simulink model "ActiveBalancer20S"  (R2021a)
settings: Solver=VariableStepAuto  StartTime=0.0  StopTime=1500  RelTol=1e-3
undefined symbols (not defined in the file): Ion, Lithium
libraries: spsSeriesRLCBranchLib x38, spsIdealSwitchLib x22, spsBatteryLib x20, spsDiodeLib x20, spsCurrentMeasurementLib x1, spsDCVoltageSourceLib x1, spsGroundLib x1, spsPWMGenerator2LevelLib x1, spspowerguiLib x1
settings Model: SimulationMode=rapid-accelerator  Creator=jafar  LastModifiedBy=jafar

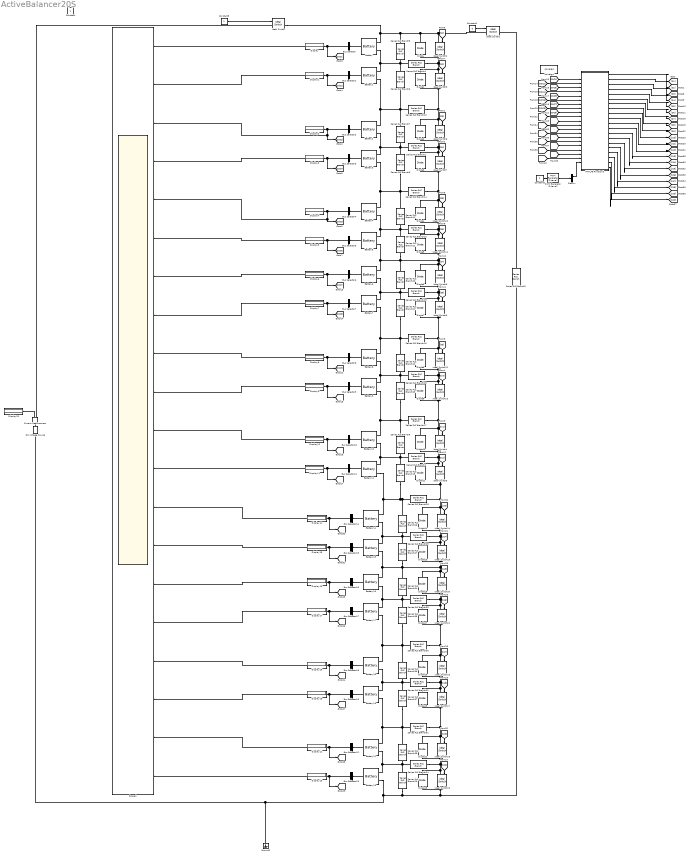
== system ActiveBalancer20S ==
  Battery : spsBatteryLib/Battery  BatType=Lithium-Ion  ShowTempParam=off  ThermalPreset=no  ShowAgeParam=off  NomV=3.7  NomQ=30  SOC=20  Batt_Tr=30  PresetModel=on  MaxQ=30  MinV=2.775  FullV=4.3068  Dis_rate=13.0435  R=0.0012333  Normal_OP=27.1304  expZone="[3.9974      1.4739]"  current=[6.5 13 32.5]  Units=Time  Tci=20  NomT=20  T2=-30  MaxQ2=4.8  FullV2=7.1  Normal_OP2=5.655  expZone2="[6.58           1]"  Rca=0.6  ti=2000  Dp=0  Neq0=0  Tsim=1e6  Ta1=25  Qeol=5.4*0.9  Reol=0.013333*1.2  Char_age=[2.3478, 3]  Dis_age=[2.3478, 10]  N1=1500  N2=10500  N3=1000  N4=1400  Ta2=45  N5=950
  Battery1 : spsBatteryLib/Battery  BatType=Lithium-Ion  ShowTempParam=off  ThermalPreset=no  ShowAgeParam=off  NomV=3.7  NomQ=30  SOC=23  Batt_Tr=30  PresetModel=on  MaxQ=30  MinV=2.775  FullV=4.3068  Dis_rate=13.0435  R=0.0012333  Normal_OP=27.1304  expZone="[3.9974      1.4739]"  current=[6.5 13 32.5]  Units=Time  Tci=20  NomT=20  T2=-30  MaxQ2=4.8  FullV2=7.1  Normal_OP2=5.655  expZone2="[6.58           1]"  Rca=0.6  ti=2000  Dp=0  Neq0=0  Tsim=1e6  Ta1=25  Qeol=5.4*0.9  Reol=0.013333*1.2  Char_age=[2.3478, 3]  Dis_age=[2.3478, 10]  N1=1500  N2=10500  N3=1000  N4=1400  Ta2=45  N5=950
  Battery10 : spsBatteryLib/Battery  BatType=Lithium-Ion  ShowTempParam=off  ThermalPreset=no  ShowAgeParam=off  NomV=3.7  NomQ=30  SOC=60  Batt_Tr=30  PresetModel=on  MaxQ=30  MinV=2.775  FullV=4.3068  Dis_rate=13.0435  R=0.0012333  Normal_OP=27.1304  expZone="[3.9974      1.4739]"  current=[6.5 13 32.5]  Units=Time  Tci=20  NomT=20  T2=-30  MaxQ2=4.8  FullV2=7.1  Normal_OP2=5.655  expZone2="[6.58           1]"  Rca=0.6  ti=2000  Dp=0  Neq0=0  Tsim=1e6  Ta1=25  Qeol=5.4*0.9  Reol=0.013333*1.2  Char_age=[2.3478, 3]  Dis_age=[2.3478, 10]  N1=1500  N2=10500  N3=1000  N4=1400  Ta2=45  N5=950
  Battery11 : spsBatteryLib/Battery  BatType=Lithium-Ion  ShowTempParam=off  ThermalPreset=no  ShowAgeParam=off  NomV=3.7  NomQ=30  SOC=63  Batt_Tr=30  PresetModel=on  MaxQ=30  MinV=2.775  FullV=4.3068  Dis_rate=13.0435  R=0.0012333  Normal_OP=27.1304  expZone="[3.9974      1.4739]"  current=[6.5 13 32.5]  Units=Time  Tci=20  NomT=20  T2=-30  MaxQ2=4.8  FullV2=7.1  Normal_OP2=5.655  expZone2="[6.58           1]"  Rca=0.6  ti=2000  Dp=0  Neq0=0  Tsim=1e6  Ta1=25  Qeol=5.4*0.9  Reol=0.013333*1.2  Char_age=[2.3478, 3]  Dis_age=[2.3478, 10]  N1=1500  N2=10500  N3=1000  N4=1400  Ta2=45  N5=950
  Battery12 : spsBatteryLib/Battery  BatType=Lithium-Ion  ShowTempParam=off  ThermalPreset=no  ShowAgeParam=off  NomV=3.7  NomQ=30  SOC=36  Batt_Tr=30  PresetModel=on  MaxQ=30  MinV=2.775  FullV=4.3068  Dis_rate=13.0435  R=0.0012333  Normal_OP=27.1304  expZone="[3.9974      1.4739]"  current=[6.5 13 32.5]  Units=Time  Tci=20  NomT=20  T2=-30  MaxQ2=4.8  FullV2=7.1  Normal_OP2=5.655  expZone2="[6.58           1]"  Rca=0.6  ti=2000  Dp=0  Neq0=0  Tsim=1e6  Ta1=25  Qeol=5.4*0.9  Reol=0.013333*1.2  Char_age=[2.3478, 3]  Dis_age=[2.3478, 10]  N1=1500  N2=10500  N3=1000  N4=1400  Ta2=45  N5=950
  Battery13 : spsBatteryLib/Battery  BatType=Lithium-Ion  ShowTempParam=off  ThermalPreset=no  ShowAgeParam=off  NomV=3.7  NomQ=30  SOC=39  Batt_Tr=30  PresetModel=on  MaxQ=30  MinV=2.775  FullV=4.3068  Dis_rate=13.0435  R=0.0012333  Normal_OP=27.1304  expZone="[3.9974      1.4739]"  current=[6.5 13 32.5]  Units=Time  Tci=20  NomT=20  T2=-30  MaxQ2=4.8  FullV2=7.1  Normal_OP2=5.655  expZone2="[6.58           1]"  Rca=0.6  ti=2000  Dp=0  Neq0=0  Tsim=1e6  Ta1=25  Qeol=5.4*0.9  Reol=0.013333*1.2  Char_age=[2.3478, 3]  Dis_age=[2.3478, 10]  N1=1500  N2=10500  N3=1000  N4=1400  Ta2=45  N5=950
  Battery14 : spsBatteryLib/Battery  BatType=Lithium-Ion  ShowTempParam=off  ThermalPreset=no  ShowAgeParam=off  NomV=3.7  NomQ=30  SOC=66  Batt_Tr=30  PresetModel=on  MaxQ=30  MinV=2.775  FullV=4.3068  Dis_rate=13.0435  R=0.0012333  Normal_OP=27.1304  expZone="[3.9974      1.4739]"  current=[6.5 13 32.5]  Units=Time  Tci=20  NomT=20  T2=-30  MaxQ2=4.8  FullV2=7.1  Normal_OP2=5.655  expZone2="[6.58           1]"  Rca=0.6  ti=2000  Dp=0  Neq0=0  Tsim=1e6  Ta1=25  Qeol=5.4*0.9  Reol=0.013333*1.2  Char_age=[2.3478, 3]  Dis_age=[2.3478, 10]  N1=1500  N2=10500  N3=1000  N4=1400  Ta2=45  N5=950
  Battery15 : spsBatteryLib/Battery  BatType=Lithium-Ion  ShowTempParam=off  ThermalPreset=no  ShowAgeParam=off  NomV=3.7  NomQ=30  SOC=69  Batt_Tr=30  PresetModel=on  MaxQ=30  MinV=2.775  FullV=4.3068  Dis_rate=13.0435  R=0.0012333  Normal_OP=27.1304  expZone="[3.9974      1.4739]"  current=[6.5 13 32.5]  Units=Time  Tci=20  NomT=20  T2=-30  MaxQ2=4.8  FullV2=7.1  Normal_OP2=5.655  expZone2="[6.58           1]"  Rca=0.6  ti=2000  Dp=0  Neq0=0  Tsim=1e6  Ta1=25  Qeol=5.4*0.9  Reol=0.013333*1.2  Char_age=[2.3478, 3]  Dis_age=[2.3478, 10]  N1=1500  N2=10500  N3=1000  N4=1400  Ta2=45  N5=950
  Battery16 : spsBatteryLib/Battery  BatType=Lithium-Ion  ShowTempParam=off  ThermalPreset=no  ShowAgeParam=off  NomV=3.7  NomQ=30  SOC=72  Batt_Tr=30  PresetModel=on  MaxQ=30  MinV=2.775  FullV=4.3068  Dis_rate=13.0435  R=0.0012333  Normal_OP=27.1304  expZone="[3.9974      1.4739]"  current=[6.5 13 32.5]  Units=Time  Tci=20  NomT=20  T2=-30  MaxQ2=4.8  FullV2=7.1  Normal_OP2=5.655  expZone2="[6.58           1]"  Rca=0.6  ti=2000  Dp=0  Neq0=0  Tsim=1e6  Ta1=25  Qeol=5.4*0.9  Reol=0.013333*1.2  Char_age=[2.3478, 3]  Dis_age=[2.3478, 10]  N1=1500  N2=10500  N3=1000  N4=1400  Ta2=45  N5=950
  Battery17 : spsBatteryLib/Battery  BatType=Lithium-Ion  ShowTempParam=off  ThermalPreset=no  ShowAgeParam=off  NomV=3.7  NomQ=30  SOC=75  Batt_Tr=30  PresetModel=on  MaxQ=30  MinV=2.775  FullV=4.3068  Dis_rate=13.0435  R=0.0012333  Normal_OP=27.1304  expZone="[3.9974      1.4739]"  current=[6.5 13 32.5]  Units=Time  Tci=20  NomT=20  T2=-30  MaxQ2=4.8  FullV2=7.1  Normal_OP2=5.655  expZone2="[6.58           1]"  Rca=0.6  ti=2000  Dp=0  Neq0=0  Tsim=1e6  Ta1=25  Qeol=5.4*0.9  Reol=0.013333*1.2  Char_age=[2.3478, 3]  Dis_age=[2.3478, 10]  N1=1500  N2=10500  N3=1000  N4=1400  Ta2=45  N5=950
  Battery18 : spsBatteryLib/Battery  BatType=Lithium-Ion  ShowTempParam=off  ThermalPreset=no  ShowAgeParam=off  NomV=3.7  NomQ=30  SOC=78  Batt_Tr=30  PresetModel=on  MaxQ=30  MinV=2.775  FullV=4.3068  Dis_rate=13.0435  R=0.0012333  Normal_OP=27.1304  expZone="[3.9974      1.4739]"  current=[6.5 13 32.5]  Units=Time  Tci=20  NomT=20  T2=-30  MaxQ2=4.8  FullV2=7.1  Normal_OP2=5.655  expZone2="[6.58           1]"  Rca=0.6  ti=2000  Dp=0  Neq0=0  Tsim=1e6  Ta1=25  Qeol=5.4*0.9  Reol=0.013333*1.2  Char_age=[2.3478, 3]  Dis_age=[2.3478, 10]  N1=1500  N2=10500  N3=1000  N4=1400  Ta2=45  N5=950
  Battery19 : spsBatteryLib/Battery  BatType=Lithium-Ion  ShowTempParam=off  ThermalPreset=no  ShowAgeParam=off  NomV=3.7  NomQ=30  SOC=33  Batt_Tr=30  PresetModel=on  MaxQ=30  MinV=2.775  FullV=4.3068  Dis_rate=13.0435  R=0.0012333  Normal_OP=27.1304  expZone="[3.9974      1.4739]"  current=[6.5 13 32.5]  Units=Time  Tci=20  NomT=20  T2=-30  MaxQ2=4.8  FullV2=7.1  Normal_OP2=5.655  expZone2="[6.58           1]"  Rca=0.6  ti=2000  Dp=0  Neq0=0  Tsim=1e6  Ta1=25  Qeol=5.4*0.9  Reol=0.013333*1.2  Char_age=[2.3478, 3]  Dis_age=[2.3478, 10]  N1=1500  N2=10500  N3=1000  N4=1400  Ta2=45  N5=950
  Battery2 : spsBatteryLib/Battery  BatType=Lithium-Ion  ShowTempParam=off  ThermalPreset=no  ShowAgeParam=off  NomV=3.7  NomQ=30  SOC=26  Batt_Tr=30  PresetModel=on  MaxQ=30  MinV=2.775  FullV=4.3068  Dis_rate=13.0435  R=0.0012333  Normal_OP=27.1304  expZone="[3.9974      1.4739]"  current=[6.5 13 32.5]  Units=Time  Tci=20  NomT=20  T2=-30  MaxQ2=4.8  FullV2=7.1  Normal_OP2=5.655  expZone2="[6.58           1]"  Rca=0.6  ti=2000  Dp=0  Neq0=0  Tsim=1e6  Ta1=25  Qeol=5.4*0.9  Reol=0.013333*1.2  Char_age=[2.3478, 3]  Dis_age=[2.3478, 10]  N1=1500  N2=10500  N3=1000  N4=1400  Ta2=45  N5=950
  Battery3 : spsBatteryLib/Battery  BatType=Lithium-Ion  ShowTempParam=off  ThermalPreset=no  ShowAgeParam=off  NomV=3.7  NomQ=30  SOC=29  Batt_Tr=30  PresetModel=on  MaxQ=30  MinV=2.775  FullV=4.3068  Dis_rate=13.0435  R=0.0012333  Normal_OP=27.1304  expZone="[3.9974      1.4739]"  current=[6.5 13 32.5]  Units=Time  Tci=20  NomT=20  T2=-30  MaxQ2=4.8  FullV2=7.1  Normal_OP2=5.655  expZone2="[6.58           1]"  Rca=0.6  ti=2000  Dp=0  Neq0=0  Tsim=1e6  Ta1=25  Qeol=5.4*0.9  Reol=0.013333*1.2  Char_age=[2.3478, 3]  Dis_age=[2.3478, 10]  N1=1500  N2=10500  N3=1000  N4=1400  Ta2=45  N5=950
  Battery4 : spsBatteryLib/Battery  BatType=Lithium-Ion  ShowTempParam=off  ThermalPreset=no  ShowAgeParam=off  NomV=3.7  NomQ=30  SOC=42  Batt_Tr=30  PresetModel=on  MaxQ=30  MinV=2.775  FullV=4.3068  Dis_rate=13.0435  R=0.0012333  Normal_OP=27.1304  expZone="[3.9974      1.4739]"  current=[6.5 13 32.5]  Units=Time  Tci=20  NomT=20  T2=-30  MaxQ2=4.8  FullV2=7.1  Normal_OP2=5.655  expZone2="[6.58           1]"  Rca=0.6  ti=2000  Dp=0  Neq0=0  Tsim=1e6  Ta1=25  Qeol=5.4*0.9  Reol=0.013333*1.2  Char_age=[2.3478, 3]  Dis_age=[2.3478, 10]  N1=1500  N2=10500  N3=1000  N4=1400  Ta2=45  N5=950
  Battery5 : spsBatteryLib/Battery  BatType=Lithium-Ion  ShowTempParam=off  ThermalPreset=no  ShowAgeParam=off  NomV=3.7  NomQ=30  SOC=45  Batt_Tr=30  PresetModel=on  MaxQ=30  MinV=2.775  FullV=4.3068  Dis_rate=13.0435  R=0.0012333  Normal_OP=27.1304  expZone="[3.9974      1.4739]"  current=[6.5 13 32.5]  Units=Time  Tci=20  NomT=20  T2=-30  MaxQ2=4.8  FullV2=7.1  Normal_OP2=5.655  expZone2="[6.58           1]"  Rca=0.6  ti=2000  Dp=0  Neq0=0  Tsim=1e6  Ta1=25  Qeol=5.4*0.9  Reol=0.013333*1.2  Char_age=[2.3478, 3]  Dis_age=[2.3478, 10]  N1=1500  N2=10500  N3=1000  N4=1400  Ta2=45  N5=950
  Battery6 : spsBatteryLib/Battery  BatType=Lithium-Ion  ShowTempParam=off  ThermalPreset=no  ShowAgeParam=off  NomV=3.7  NomQ=30  SOC=48  Batt_Tr=30  PresetModel=on  MaxQ=30  MinV=2.775  FullV=4.3068  Dis_rate=13.0435  R=0.0012333  Normal_OP=27.1304  expZone="[3.9974      1.4739]"  current=[6.5 13 32.5]  Units=Time  Tci=20  NomT=20  T2=-30  MaxQ2=4.8  FullV2=7.1  Normal_OP2=5.655  expZone2="[6.58           1]"  Rca=0.6  ti=2000  Dp=0  Neq0=0  Tsim=1e6  Ta1=25  Qeol=5.4*0.9  Reol=0.013333*1.2  Char_age=[2.3478, 3]  Dis_age=[2.3478, 10]  N1=1500  N2=10500  N3=1000  N4=1400  Ta2=45  N5=950
  Battery7 : spsBatteryLib/Battery  BatType=Lithium-Ion  ShowTempParam=off  ThermalPreset=no  ShowAgeParam=off  NomV=3.7  NomQ=30  SOC=51  Batt_Tr=30  PresetModel=on  MaxQ=30  MinV=2.775  FullV=4.3068  Dis_rate=13.0435  R=0.0012333  Normal_OP=27.1304  expZone="[3.9974      1.4739]"  current=[6.5 13 32.5]  Units=Time  Tci=20  NomT=20  T2=-30  MaxQ2=4.8  FullV2=7.1  Normal_OP2=5.655  expZone2="[6.58           1]"  Rca=0.6  ti=2000  Dp=0  Neq0=0  Tsim=1e6  Ta1=25  Qeol=5.4*0.9  Reol=0.013333*1.2  Char_age=[2.3478, 3]  Dis_age=[2.3478, 10]  N1=1500  N2=10500  N3=1000  N4=1400  Ta2=45  N5=950
  Battery8 : spsBatteryLib/Battery  BatType=Lithium-Ion  ShowTempParam=off  ThermalPreset=no  ShowAgeParam=off  NomV=3.7  NomQ=30  SOC=54  Batt_Tr=30  PresetModel=on  MaxQ=30  MinV=2.775  FullV=4.3068  Dis_rate=13.0435  R=0.0012333  Normal_OP=27.1304  expZone="[3.9974      1.4739]"  current=[6.5 13 32.5]  Units=Time  Tci=20  NomT=20  T2=-30  MaxQ2=4.8  FullV2=7.1  Normal_OP2=5.655  expZone2="[6.58           1]"  Rca=0.6  ti=2000  Dp=0  Neq0=0  Tsim=1e6  Ta1=25  Qeol=5.4*0.9  Reol=0.013333*1.2  Char_age=[2.3478, 3]  Dis_age=[2.3478, 10]  N1=1500  N2=10500  N3=1000  N4=1400  Ta2=45  N5=950
  Battery9 : spsBatteryLib/Battery  BatType=Lithium-Ion  ShowTempParam=off  ThermalPreset=no  ShowAgeParam=off  NomV=3.7  NomQ=30  SOC=57  Batt_Tr=30  PresetModel=on  MaxQ=30  MinV=2.775  FullV=4.3068  Dis_rate=13.0435  R=0.0012333  Normal_OP=27.1304  expZone="[3.9974      1.4739]"  current=[6.5 13 32.5]  Units=Time  Tci=20  NomT=20  T2=-30  MaxQ2=4.8  FullV2=7.1  Normal_OP2=5.655  expZone2="[6.58           1]"  Rca=0.6  ti=2000  Dp=0  Neq0=0  Tsim=1e6  Ta1=25  Qeol=5.4*0.9  Reol=0.013333*1.2  Char_age=[2.3478, 3]  Dis_age=[2.3478, 10]  N1=1500  N2=10500  N3=1000  N4=1400  Ta2=45  N5=950
  Bus Selector{,1..19} (20 alike) : BusSelector  OutputSignals=SOC (%)
  Constant1 : Constant  Value=0
  Constant2 : Constant  Value=2
  Constant5 : Constant
  Current Measurement : spsCurrentMeasurementLib/Current Measurement  PhasorSimulation=off  OutputType=Complex  PSBequivalent=0
  DC Voltage Source : spsDCVoltageSourceLib/DC Voltage Source  Amplitude=84  Measurements=None
  Demux : Demux  Outputs=2
  Diode{,1..19} (20 alike) : spsDiodeLib/Diode  Ron=0.001  Lon=0  Vf=0.8  IC=0  UseSnubber=0  Rs=500  Cs=250e-9  Measurements=off
  Display{,1..20} (21 alike) : Display
  Ground1 : spsGroundLib/Ground  LConnTagsString=a
  Ideal Switch : spsIdealSwitchLib/Ideal Switch  Ron=0.001  Lon=0  IC=0  Rs=1e5  Cs=inf  Measurements=on
  Ideal Switch1 : spsIdealSwitchLib/Ideal Switch  Ron=0.001  Lon=0  IC=0  Rs=1e5  Cs=inf  Measurements=on
  Ideal Switch{2..21} (20 alike) : spsIdealSwitchLib/Ideal Switch  Ron=0.001  Lon=0  IC=0  Rs=1e5  Cs=inf  Measurements=off
  MATLAB Function3 : MATLAB Function  TreatAsAtomicUnit=on
  PWM Generator (2-Level) : spsPWMGenerator2LevelLib/PWM Generator (2-Level)  ModulatorType=Single-phase half-bridge (2 pulses)  ModulatorMode=Unsynchronized  Fc=500  Pc=0  nF=27  MinMax="[ -1  1 ]"  SamplingTechnique=Natural  ModulatingSignals=off  m=0.8  Freq=60  Phase=0  Ts=0  ShowCarrierOutport=off
  Scope1 : Scope  NumInputPorts=20
  Series RLC Branch{1..2,4,10,13..14,16..19,24..25,28,30..33} (17 alike) : spsSeriesRLCBranchLib/Series RLC Branch  LConnTagsString=__new0  RConnTagsString=__new0  BranchType=L  Resistance=1  Inductance=1e-3  SetiL0=off  InitialCurrent=0  Capacitance=1e-6  Setx0=off  InitialVoltage=0  Measurements=None
  Series RLC Branch{5..9,11..12,15,20..23,26..27,29,34..38} (20 alike) : spsSeriesRLCBranchLib/Series RLC Branch  LConnTagsString=__new0  RConnTagsString=__new0  BranchType=C  Resistance=1  Inductance=1e-3  SetiL0=off  InitialCurrent=0  Capacitance=1e-6  Setx0=off  InitialVoltage=0  Measurements=None
  Series RLC Branch3 : spsSeriesRLCBranchLib/Series RLC Branch  LConnTagsString=__new0  RConnTagsString=__new0  BranchType=R  Resistance=1.73  Inductance=1e-3  SetiL0=off  InitialCurrent=0  Capacitance=1e-6  Setx0=off  InitialVoltage=0  Measurements=None
  powergui : spspowerguiLib/powergui  Priority=1  SimulationMode=Discrete  SampleTime=50e-5  frequency=60  Iterations=50  frequencyindice=0  Pbase=100e6  ErrMax=1e-4  UnitsV=kV  UnitsW=MW  buscounter=0  FunctionMessages=off  echomessages=off  EnableUseOfTLC=off  CurrentSourceSwitches=off  DisableSnubberDevices=off  DisableRonSwitches=off  DisableVfSwitches=off  DisplayEquations=off  AutomaticDiscreteSolvers=off  SolverType=Tustin/Backward Euler (TBE)  Interpol=off  ExternalGateDelay=off  methode=off  Ts=100  x0status=blocks  SPID=on  SwTol=0  HookPort=off  NonlinearTolerance=1e-4  nMaxIteration=100  ContinueOnMaxIteration=off  RestoreLinks=warning  ResistiveCurrentMeasurement=off  Frange=[0:2:500]  Ylog=off  Xlog=on  ShowGrid=off  save=off  variable=ZData  structure=0  ZoomFFT=off  StartTime=0.0  cycles=1  DisplayStyle=1  fundamental=60  FreqAxis=off  MaxFrequency=1000  frequencyindicesteady=1  RmsSteady=1  display=off
  Constant : Constant  IOType=siggen
  wires:
  MATLAB Function3/9(S9) -> [S9]
  [SOC8] -> MATLAB Function3/8(SOC8)
  Battery4/1 -> Bus Selector4/1
  Bus Selector9/1 -> Scope1/10, [SOC10], Display9/1  "<SOC (%)>"
  [S7] -> Ideal Switch8/1
  Demux/1 -> MATLAB Function3/21(PWM)
  [SOC6] -> MATLAB Function3/6(SOC6)
  PWM Generator (2-Level)/1 -> Demux/1
  Bus Selector8/1 -> Scope1/9, [SOC9], Display8/1  "<SOC (%)>"
  Battery11/1 -> Bus Selector11/1
  [SOC3] -> MATLAB Function3/3(SOC3)
  [SOC7] -> MATLAB Function3/7(SOC7)
  MATLAB Function3/11(S11) -> [S11]
  Battery5/1 -> Bus Selector5/1
  Battery10/1 -> Bus Selector10/1
  MATLAB Function3/10(S10) -> [S10]
  [SOC11] -> MATLAB Function3/11(SOC11)
  Battery9/1 -> Bus Selector9/1
  [S12] -> Ideal Switch5/1
  [S10] -> Ideal Switch13/1
  [SOC2] -> MATLAB Function3/2(SOC2)
  [S8] -> Ideal Switch9/1
  [SOC10] -> MATLAB Function3/10(SOC10)
  Battery7/1 -> Bus Selector7/1
  Battery8/1 -> Bus Selector8/1
  [S1] -> Ideal Switch2/1
  [SOC12] -> MATLAB Function3/12(SOC12)
  Bus Selector11/1 -> Scope1/12, [SOC12], Display11/1  "<SOC (%)>"
  [S3] -> Ideal Switch6/1
  [SOC4] -> MATLAB Function3/4(SOC4)
  Bus Selector6/1 -> Scope1/7, [SOC7], Display6/1  "<SOC (%)>"
  MATLAB Function3/1(S1) -> [S1]
  Bus Selector10/1 -> Scope1/11, [SOC11], Display10/1  "<SOC (%)>"
  Bus Selector2/1 -> [SOC3], Scope1/3, Display2/1  "<SOC (%)>"
  Constant5/1 -> Ideal Switch/1
  MATLAB Function3/8(S8) -> [S8]
  Constant1/1 -> Ideal Switch1/1
  Battery1/1 -> Bus Selector1/1
  Bus Selector1/1 -> Scope1/2, [SOC2], Display1/1  "<SOC (%)>"
  Bus Selector7/1 -> Scope1/8, [SOC8], Display7/1  "<SOC (%)>"
  MATLAB Function3/12(S12) -> [S12]
  MATLAB Function3/5(S5) -> [S5]
  Constant2/1 -> PWM Generator (2-Level)/1
  [S11] -> Ideal Switch4/1
  [SOC5] -> MATLAB Function3/5(SOC5)
  [SOC1] -> MATLAB Function3/1(SOC1)
  MATLAB Function3/7(S7) -> [S7]
  MATLAB Function3/2(S2) -> [S2]
  Battery3/1 -> Bus Selector3/1
  Battery/1 -> Bus Selector/1
  [S2] -> Ideal Switch3/1
  Bus Selector/1 -> Scope1/1, [SOC1], Display/1  "<SOC (%)>"
  [S4] -> Ideal Switch7/1
  [S6] -> Ideal Switch11/1
  [S5] -> Ideal Switch10/1
  Battery2/1 -> Bus Selector2/1
  MATLAB Function3/6(S6) -> [S6]
  MATLAB Function3/3(S3) -> [S3]
  Bus Selector3/1 -> Scope1/4, [SOC4], Display3/1  "<SOC (%)>"
  Bus Selector5/1 -> Scope1/6, [SOC6], Display5/1  "<SOC (%)>"
  Bus Selector4/1 -> Scope1/5, [SOC5], Display4/1  "<SOC (%)>"
  [SOC9] -> MATLAB Function3/9(SOC9)
  [S9] -> Ideal Switch12/1
  Battery6/1 -> Bus Selector6/1
  MATLAB Function3/4(S4) -> [S4]
  Battery14/1 -> Bus Selector14/1
  [S17] -> Ideal Switch16/1
  Battery16/1 -> Bus Selector16/1
  Bus Selector15/1 -> Scope1/14, [SOC14], Display15/1  "<SOC (%)>"
  [S14] -> Ideal Switch15/1
  [S19] -> Ideal Switch18/1
  Bus Selector17/1 -> Scope1/16, [SOC16], Display17/1  "<SOC (%)>"
  Bus Selector16/1 -> Scope1/15, [SOC15], Display16/1  "<SOC (%)>"
  Bus Selector13/1 -> Scope1/20, [SOC20], Display13/1  "<SOC (%)>"
  Battery13/1 -> Bus Selector13/1
  Battery18/1 -> Bus Selector18/1
  Bus Selector14/1 -> Scope1/13, [SOC13], Display14/1  "<SOC (%)>"
  Bus Selector18/1 -> Scope1/17, [SOC17], Display18/1  "<SOC (%)>"
  [S13] -> Ideal Switch14/1
  [S20] -> Ideal Switch19/1
  Battery15/1 -> Bus Selector15/1
  Battery12/1 -> Bus Selector12/1
  Battery19/1 -> Bus Selector19/1
  Battery17/1 -> Bus Selector17/1
  [S18] -> Ideal Switch17/1
  [S15] -> Ideal Switch20/1
  Bus Selector19/1 -> Scope1/18, [SOC18], Display19/1  "<SOC (%)>"
  [S16] -> Ideal Switch21/1
  Bus Selector12/1 -> Scope1/19, [SOC19], Display12/1  "<SOC (%)>"
  [SOC18] -> MATLAB Function3/18(SOC18)
  [SOC19] -> MATLAB Function3/19(SOC19)
  [SOC14] -> MATLAB Function3/14(SOC14)
  [SOC20] -> MATLAB Function3/20(SOC20)
  [SOC13] -> MATLAB Function3/13(SOC13)
  [SOC16] -> MATLAB Function3/16(SOC16)
  [SOC15] -> MATLAB Function3/15(SOC15)
  [SOC17] -> MATLAB Function3/17(SOC17)
  MATLAB Function3/19(S19) -> [S19]
  MATLAB Function3/14(S14) -> [S14]
  MATLAB Function3/16(S16) -> [S16]
  MATLAB Function3/15(S15) -> [S15]
  MATLAB Function3/17(S17) -> [S17]
  MATLAB Function3/18(S18) -> [S18]
  MATLAB Function3/13(S13) -> [S13]
  MATLAB Function3/20(S20) -> [S20]
  Current Measurement/1 -> Display20/1
  connections:
  Series RLC Branch19/RConn1 -- Ideal Switch8/RConn1 -- Diode6/LConn1 -- Diode7/RConn1 -- Ideal Switch9/LConn1
  Battery8/LConn1 -- Series RLC Branch16/LConn1 -- Series RLC Branch22/LConn1 -- Series RLC Branch21/RConn1 -- Battery7/LConn2
  Series RLC Branch9/RConn1 -- Series RLC Branch1/LConn1 -- Series RLC Branch15/LConn1 -- Battery10/LConn2 -- Battery11/LConn1
  Series RLC Branch22/RConn1 -- Battery8/LConn2 -- Battery9/LConn1 -- Series RLC Branch18/LConn1 -- Series RLC Branch23/LConn1
  Battery13/LConn2 -- Series RLC Branch3/RConn1 -- Diode13/LConn1 -- Ideal Switch19/RConn1 -- Series RLC Branch29/RConn1 -- DC Voltage Source/LConn1 -- Ground1/LConn1
  Ideal Switch4/LConn1 -- Diode10/RConn1 -- Series RLC Branch17/RConn1 -- Diode9/LConn1 -- Ideal Switch13/RConn1
  Diode2/LConn1 -- Series RLC Branch2/RConn1 -- Ideal Switch7/LConn1 -- Diode3/RConn1 -- Ideal Switch6/RConn1
  Battery7/LConn1 -- Series RLC Branch20/RConn1 -- Series RLC Branch19/LConn1 -- Series RLC Branch21/LConn1 -- Battery6/LConn2
  Ideal Switch4/RConn1 -- Diode11/RConn1 -- Ideal Switch5/LConn1 -- Series RLC Branch1/RConn1 -- Diode10/LConn1
  Series RLC Branch13/LConn1 -- Series RLC Branch7/LConn1 -- Series RLC Branch6/RConn1 -- Battery1/LConn2 -- Battery2/LConn1
  Series RLC Branch8/RConn1 -- Battery3/LConn2 -- Battery4/LConn1 -- Series RLC Branch14/LConn1 -- Series RLC Branch11/LConn1
  Diode3/LConn1 -- Ideal Switch7/RConn1 -- Series RLC Branch14/RConn1 -- Diode4/RConn1 -- Ideal Switch10/LConn1
  Battery4/LConn2 -- Battery5/LConn1 -- Series RLC Branch10/LConn1 -- Series RLC Branch12/LConn1 -- Series RLC Branch11/RConn1
  Diode8/LConn1 -- Ideal Switch12/RConn1 -- Diode9/RConn1 -- Ideal Switch13/LConn1 -- Series RLC Branch18/RConn1
  Series RLC Branch10/RConn1 -- Diode4/LConn1 -- Ideal Switch10/RConn1 -- Ideal Switch11/LConn1 -- Diode5/RConn1
  Battery2/LConn2 -- Battery3/LConn1 -- Series RLC Branch2/LConn1 -- Series RLC Branch8/LConn1 -- Series RLC Branch7/RConn1
  Battery1/LConn1 -- Series RLC Branch4/LConn1 -- Series RLC Branch6/LConn1 -- Series RLC Branch5/RConn1 -- Battery/LConn2
  Diode1/RConn1 -- Ideal Switch3/LConn1 -- Ideal Switch2/RConn1 -- Diode/LConn1 -- Series RLC Branch4/RConn1
  Ideal Switch9/RConn1 -- Series RLC Branch16/RConn1 -- Diode8/RConn1 -- Ideal Switch12/LConn1 -- Diode7/LConn1
  Diode5/LConn1 -- Ideal Switch11/RConn1 -- Battery5/LConn2 -- Battery6/LConn1 -- Series RLC Branch20/LConn1 -- Series RLC Branch12/RConn1 -- Diode6/RConn1 -- Ideal Switch8/LConn1
  Series RLC Branch9/LConn1 -- Series RLC Branch23/RConn1 -- Battery9/LConn2 -- Battery10/LConn1 -- Series RLC Branch17/LConn1
  Ideal Switch6/LConn1 -- Diode1/LConn1 -- Ideal Switch3/RConn1 -- Series RLC Branch13/RConn1 -- Diode2/RConn1
  Series RLC Branch5/LConn1 -- Diode/RConn1 -- Ideal Switch2/LConn1 -- Ideal Switch1/LConn1 -- Battery/LConn1 -- Ideal Switch/RConn1
  Ideal Switch/LConn1 -- Current Measurement/RConn1
  Series RLC Branch3/LConn1 -- Ideal Switch1/RConn1
  Ideal Switch21/RConn1 -- Series RLC Branch30/RConn1 -- Diode18/RConn1 -- Ideal Switch16/LConn1 -- Diode17/LConn1
  Series RLC Branch25/RConn1 -- Diode14/LConn1 -- Ideal Switch14/RConn1 -- Diode15/RConn1 -- Ideal Switch15/LConn1
  Series RLC Branch38/LConn1 -- Series RLC Branch37/RConn1 -- Series RLC Branch31/LConn1 -- Battery19/LConn2 -- Battery12/LConn1
  Diode15/LConn1 -- Ideal Switch15/RConn1 -- Diode16/RConn1 -- Ideal Switch20/LConn1 -- Battery15/LConn2 -- Battery16/LConn1 -- Series RLC Branch34/LConn1 -- Series RLC Branch27/RConn1
  Diode18/LConn1 -- Ideal Switch16/RConn1 -- Series RLC Branch32/RConn1 -- Diode19/RConn1 -- Ideal Switch17/LConn1
  Battery14/LConn2 -- Series RLC Branch25/LConn1 -- Series RLC Branch27/LConn1 -- Series RLC Branch26/RConn1 -- Battery15/LConn1
  Ideal Switch18/RConn1 -- Diode12/LConn1 -- Series RLC Branch24/RConn1 -- Diode13/RConn1 -- Ideal Switch19/LConn1
  Battery17/LConn1 -- Battery16/LConn2 -- Series RLC Branch34/RConn1 -- Series RLC Branch33/LConn1 -- Series RLC Branch35/LConn1
  Ideal Switch18/LConn1 -- Diode12/RConn1 -- Series RLC Branch31/RConn1 -- Diode19/LConn1 -- Ideal Switch17/RConn1
  Series RLC Branch38/RConn1 -- Series RLC Branch24/LConn1 -- Series RLC Branch29/LConn1 -- Battery12/LConn2 -- Battery13/LConn1
  Series RLC Branch36/RConn1 -- Series RLC Branch32/LConn1 -- Series RLC Branch37/LConn1 -- Battery18/LConn2 -- Battery19/LConn1
  Battery18/LConn1 -- Battery17/LConn2 -- Series RLC Branch30/LConn1 -- Series RLC Branch36/LConn1 -- Series RLC Branch35/RConn1
  Series RLC Branch26/LConn1 -- Series RLC Branch15/RConn1 -- Battery11/LConn2 -- Battery14/LConn1 -- Series RLC Branch28/LConn1
  Series RLC Branch33/RConn1 -- Ideal Switch20/RConn1 -- Diode16/LConn1 -- Diode17/RConn1 -- Ideal Switch21/LConn1
  Ideal Switch14/LConn1 -- Diode14/RConn1 -- Diode11/LConn1 -- Ideal Switch5/RConn1 -- Series RLC Branch28/RConn1
  DC Voltage Source/RConn1 -- Current Measurement/LConn1

== matlab function ActiveBalancer20S/MATLAB Function3 ==
  data: SOC1 input; S1 output; SOC2 input; SOC3 input; SOC4 input; SOC5 input; SOC6 input; SOC7 input; SOC8 input; SOC9 input; SOC10 input; SOC11 input; SOC12 input; SOC13 input; SOC14 input; SOC15 input; SOC16 input; SOC17 input; SOC18 input; SOC19 input; SOC20 input; S2 output; S3 output; S4 output; S5 output; S6 output; PWM input; S7 output; S8 output; S9 output; S10 output; S11 output; S12 output; S13 output; S14 output; S15 output; S16 output; S17 output; S18 output; S19 output; S20 output
function [S1, S2, S3, S4, S5, S6, S7, S8, S9, S10, S11, S12, S13, S14, S15, S16, S17, S18, S19, S20] = fcn(SOC1, SOC2, SOC3, SOC4, SOC5, SOC6, SOC7, SOC8, SOC9, SOC10, SOC11, SOC12, SOC13, SOC14, SOC15, SOC16, SOC17, SOC18, SOC19, SOC20, PWM)
    datas = [SOC1, SOC2, SOC3, SOC4, SOC5, SOC6, SOC7, SOC8, SOC9, SOC10, SOC11, SOC12, SOC13, SOC14, SOC15, SOC16, SOC17, SOC18, SOC19, SOC20];
    output = zeros(size(datas));
    rata_rata = mean(datas);
    
    for i = 1:length(datas)
        if datas(i) > rata_rata
            output(i) = PWM;
        else
            output(i) = 0;
        end
    end
    
    S1 = output(1);
    S2 = output(2);
    S3 = output(3);
    S4 = output(4);
    S5 = output(5);
    S6 = output(6);
    S7 = output(7);
    S8 = output(8);
    S9 = output(9);
    S10 = output(10);
    S11 = output(11);
    S12 = output(12);
    S13 = output(13);
    S14 = output(14);
    S15 = output(15);
    S16 = output(16);
    S17 = output(17);
    S18 = output(18);
    S19 = output(19);
    S20 = output(20);
end
